simulink library "NCS_Library"  (R2019a)
settings: Solver=VariableStepAuto  StartTime=0.0  StopTime=10.0  RelTol=1e-3
values from neighbouring files (symbols this model uses):
  A = 10    [Parameter.m]
  band = 100000000    [Parameter.m]
  BER = 0    [Parameter.m]
  c = 5000000    [Parameter.m]
  c1 = 4.33    [Parameter.m]
  c2 = 3.16    [Parameter.m]
  CAN2EthernetDelay = 0.000    (= 0)    [Parameter.m]
  cR = 1.5*10^-3    (= 0.0015)    [Parameter.m]
  cw = (cwE * 2 + cwM * (nW_ges-2))/nW_ges    (= 0.1475)    [Parameter.m]
  cwE = 0.35    [Parameter.m]
  cwM = 0.08    [Parameter.m]
  Cycle_Controller = 0    [Parameter.m]
  CyclePLC = 24/1000    (= 0.024)    [Parameter.m]
  d = 800000    [Parameter.m]
  Dr = 0.92    [Parameter.m]
  Ethernet2CANDelay = 0.005    [Parameter.m]
  F_konst = 70892    [Parameter.m]
  FA = 100000    [Parameter.m]
  FB_WB_max = 10000    [Parameter.m]
  FBel_an = iG*nG*F_KZmax*nBan*R_mR/(Dr/2)    (= 28197.4297239)    [Parameter.m]
  FBel_frei = iG*nG*F_KZmax*nBfrei*R_mW/(Dr/2)    (= 29270.6882948)    [Parameter.m]
  Fmaxdyn = 300000    [Parameter.m]
  g = 9.81    [Parameter.m]
  i = 0    [Parameter.m]
  J = 1/2*mA*(Dr/2)^2    (= 158.7)    [Parameter.m]
  k1 = 0.095    [Parameter.m]
  k2 = 9.26/3.6    (= 2.57222222222)    [Parameter.m]
  k3 = 4.63/3.6    (= 1.28611111111)    [Parameter.m]
  mges = 58000    [Parameter.m]
  mu = [mu1 mu2]    [Parameter.m]
  muBel1 = 0.42    [Parameter.m]
  muBel2 = 0.36    [Parameter.m]
  n = 0.001    [Parameter.m]
  n_Mg = 4    [Parameter.m]
  n_WB = 4    [Parameter.m]
  nA = 4    [Parameter.m]
  nBan = 2    [Parameter.m]
  nBfrei = 3    [Parameter.m]
  nM = 4    [Parameter.m]
  nW_an = 4    [Parameter.m]
  P_max = 8200000    [Parameter.m]
  Q = 10    [Parameter.m]
  r_reib = 600    [Parameter.m]
  rho = 1.08    [Parameter.m]
  rhoL = 1.225    [Parameter.m]
  Size = 8    [Parameter.m]
  slip = [s1 s2]    [Parameter.m]
  tol = 0.05    [Parameter.m]
  v00 = 100/3.6    (= 27.7777777778)    [Parameter.m]
  v_grenz = 60/3.6    (= 16.6666666667)    [Parameter.m]
  v_opt = 75/3.6    (= 20.8333333333)    [Parameter.m]
  W_opt = 0.5    [Parameter.m]
  WB = 1    [Parameter.m]
  y_opt = sqrt(W_opt)/((1+sqrt(W_opt))^2+W_opt)    [Parameter.m]
undefined symbols (not defined in the file or in its folder): BUSCapacity, CableLength, controlGate, D_dyn, D_mg, EnableBurst, EnableToF, entity, Entity_out, Gate, Gate_4, Gate_5, Gate_ACK, Gate_copy, Gate_RX, getData, gettime, I_dyn, I_mg, m, magnitude, P_dyn, P_mg, ReadAttributes, readdata, ReadData, ReadSize, sigbuilder_block, Timeout, ToB, ToF, v0, v_d, v_soll
libraries: simulink x176, $bdroot x102
(part 11 of 12)

== matlab function NCS_Library/Network/ETB/OSI Layers/IP/Simulink Function/MATLAB Function ==
  data: Source input; Destination input; MACSource output; MACDestination output
function [ MACSource, MACDestination ] = GetMAC( Source, Destination)
% This function determnines if the the destination of the entity is of
% the same consist or of a remote consist.
% If it is in a remote consist, the entity is sent to the TBN/router.
if Source(1) == Destination(1)
    MACDestination = uint16(Destination(2));
elseif Destination(1) == 100
    % Multicast
    MACDestination = uint16(200);
else
    MACDestination = uint16(99);
    % to router
end
MACSource = Source(2);
end % end function

== stateflow chart NCS_Library/Network/Gateway/Gateway1/CAN Interface/CAN Interface/Reception Control ==
  settings: enableNonTerminalStates=1
  state Process
    en:
    Port.data=S;
    send(Port);
  state [Status,Ack] = Compute(rx_id,loss,rx_rtr,rx_data,tx_id,tx_rtr,tx_data) [function]
  (default) -> Process : {S=1; Ack=0; TX_ID=-1; TX_RTR=0; TX_Data=0;}
  Process -> Process [order 1] : TX{TX_ID=TX.data.ID; TX_RTR=TX.data.RTR; TX_Data=TX.data.Data;}
  (junction 12) -> Process [order 1] : [Ack==1]{Success.data=1; send(Success);}
  (junction 12) -> Process [order 2] : [Ack==0]{ReTX.data=1; send(ReTX);}
  Process -> (junction 12) [order 2] : RX{[S,Ack]=Compute(RX.data.ID,...
      |                         RX.data.RndLoss, ...
      |                         RX.data.RTR, ...
      |                         RX.data.Data, ...
      |                         TX_ID, ...
      |                         TX_RTR, ...
      |                         TX_Data);}
  data: Status function_output; Ack function_output; rx_id function_input double size=1; loss function_input double size=1; rx_rtr function_input double size=1; rx_data function_input double size=1; tx_id function_input double size=1; tx_rtr function_input double size=1; tx_data function_input double size=1; TX input Bus: CAN_Message; RX input Bus: CAN_Message; S local; Ack local; TX_ID local; TX_RTR local; TX_Data local; Port output; Success output; ReTX output

== matlab function NCS_Library/Network/Gateway/Gateway1/CAN Interface/CAN Interface/Reception Control/Compute/MATLAB Function ==
  data: ID0 input; ACK output; RTR0 input; Data0 input; ID1 input; RTR1 input; Data1 input; Loss input
function ACK = fcn(ID0,RTR0,Data0,ID1,RTR1,Data1,Loss)
% Compare the message ID, RTR, Data fields to acknowledge a successful send

if (ID0 == ID1 && RTR0 == RTR1 && Data0 == Data1 && Loss < 1)
    ACK = 1;
else
    ACK = 0;
end

== stateflow chart NCS_Library/Network/Gateway/Gateway1/CAN Interface/Save Data/Hold Data ==
  state Init
    en: SavedData=InData;
  state Save_Data
    du: OutData=SavedData;
  state Push_Data
    en: OutData=SavedData;
  (default) -> Init
  Init -> Save_Data
  Push_Data -> Save_Data
  Save_Data -> Push_Data : [Flush==1]{SavedData=InData;}
  data: Flush input; InData input; SavedData local; OutData output

== matlab function NCS_Library/Network/Gateway/Gateway1/CAN Interface/Save Data/MATLAB Function ==
  data: refresh input; write input; Type input; Data input; M_Data output; M_Data_old input
function M_Data = SaveData (refresh, write, Type, Data, M_Data_old)
%% Init
M_Data = zeros(3,20);
M_Data(1,1) = 1;

if refresh
    % refresh matrix
else
    % save data in matrix
    M_Data = M_Data_old;
    if write && Type > 0 && Type < 3
        if M_Data(1,1) == 1
            % no data saved yet
            M_Data(Type,2) = Data;          % save data
            M_Data(1,1) = M_Data(1,1)+1;    % update length
        else
            % compare the data to write with the data already saved in the matrix
            for i=2:M_Data(1,1)+1
                if M_Data(1,i) ~= 0 || M_Data(2,i) ~= 0 || M_Data(3,i) ~= 0
                    % there is data at current position
                    if M_Data(Type,i) == Data
                        % data on current position is data to write
                        break;  % data already saved in Ethernet entity
                    end
                else
                    M_Data(Type,i) = Data;          % save data
                    M_Data(1,1) = M_Data(1,1)+1;    % update length
                    break;  % finished
                end
            end % endfor
        end
    end %endif write
end % endif refresh
end % function

== matlab function NCS_Library/Network/ETB/OSI Layers/IP/Simulink Function1/MATLAB Function ==
  data: Address input; Route output; Source input; Destination input; SN input
function Route = Addressing(Address, Source, Destination, SN)
%% This function determines if the incoming entity is a mulitcast of a subscribed node
% It checks if there is a multicast and if the source is a subscribed node.
% Depending on that, the route is chosen.
%% Init
Route = uint8(2);
s = size(SN);
%% get route
if Destination(1) < 100
    % invalid address
    Route = uint8(2);   % discard
elseif Destination(1) == Address(1)
    if Destination(2) == 200
        % Broadcast to Consist
        Route = uint8(2);
        for i=1:s(2)
            if Source(1) == SN(i,1) && Source(2) == SN(i,2) && Source(3) == SN(i,3) && Source(4) == SN(i,4)
                % subscribed to node
                Route = uint8(1);  
                break;
            end
        end
    elseif Destination(4) == Address(4)
            Route = uint8(1);  % set route
    else
        Route = uint8(2);   % discard
    end
elseif Destination(1) == 100
    % Multicast
    Route = uint8(2);
    for i=1:s(2)
        if Source(1) == SN(i,1) && Source(2) == SN(i,2) && Source(3) == SN(i,3) && Source(4) == SN(i,4)
            % subscribed to node
            Route = uint8(1);  
            break;
        end
    end
else
    Route = uint8(2);   % discard
end % endif
end % end function

== matlab function NCS_Library/Network/ETB/OSI Layers/TRDP PD/Simulink Function1/MATLAB Function2 ==
  data: msgType input; ReplyAddress input; DestinationPull output
function DestinationPull = Receive(msgType, ReplyAddress)

DestinationPull = uint16( [0 0 0 0] );

if msgType == 11
    % Request
    DestinationPull = ReplyAddress;
end
        
end % end function

== matlab function NCS_Library/Network/ETB/OSI Layers/TRDP PD/Simulink Function/MATLAB Function ==
  data: Data input; Data_edited output; msgType input
function Data_edited = EditData(Data, msgType)
%% Edit Data
% Replace data with zero in the case of a request or an error.

if msgType == 11 || msgType == 14
    Data_edited = zeros(3, 20);
else
    Data_edited = Data;
end

end % end of function

== matlab function NCS_Library/Network/ETB/OSI Layers/SDTv2/MATLAB Function ==
  data: T_signal input; msgType input; y output; T_tx input
function y = fcn(T_signal, msgType, T_tx)

if msgType == 11
    y = T_signal;
else
    y = T_tx;
end
end

== matlab function NCS_Library/Network/ETB/OSI Layers/SDTv2/Simulink Function1/MATLAB Function ==
  data: SSC_received output; SSC_last input; SSC input; Route output
function [ SSC_received , Route]= Check( SSC_last, SSC)
%% Check the SSC of the VDP
% This functions checks the SSC of an arriving VDP. If the SSC is greater
% or equal to SSC of the last fresh VDP received the VDP is valid. If it is
% greater than the last, the VDP is fresh and its SSC is saved.

Route = uint8(2); % discard for default
SSC_received = SSC_last;

if SSC > SSC_last
    Route = uint8(1);
    SSC_received = SSC;
elseif SSC == 0
    % Init
    Route = uint8(1);
end

== matlab function NCS_Library/Network/ETB/Controller Interface/Parameter/MATLAB Function ==
  data: In1 input; In2 input; msgType output; In3 input; In4 input
function msgType = GetmsgType(In1, In2, In3, In4)

In = [In1 In2 In3 In4];

n = length(In);
msgType = uint8(zeros(n,1));   % Init

for i=1:n
    if In(i) == 1
        % Push Data
        Type = 13;
    else
        Type = 0;
    end
    msgType(i) = uint8(Type);
end
end % end function

== matlab function NCS_Library/Network/ETB/OSI Layers/SDTv2/Get Phase/MATLAB Function ==
  data: Phase_previous input; LSC input; Phase output; Contraction input; Init input
function Phase = Get_SDTv2_Phase(Phase_previous, LSC, Contraction, Init)
%% This function determines the phase of the SDTv2
% Phase 0: no inital VDP sampled
% Phase 1: Safe
% Phase 2: Sink-Time error
% Phase 3: Contraction
%% Set Phase
Phase = Phase_previous;

switch Phase
    case 0
        % No received inital VDP
        if Init
            Phase = 1;
        else
            Phase = 0;
        end
    case 1
        % Safe communication
        if LSC
            Phase = 2;
        elseif Contraction
            Phase = 3;
        else
            Phase = 1;
        end
    case 2
        % Lost of safe communication
        if ~LSC
            Phase = 1;
        end
    case 3
        if ~Contraction
            Phase = 1;
        end
    otherwise
        Phase = 10;
end
end % end function

== matlab function NCS_Library/Network/ETB/Controller Interface/Parameter/MATLAB Function1 ==
  data: Destination output; Actuators input; Sensors input; Subscribe output
function [ Destination, Subscribe]= AddMatrices(Actuators, Sensors)

Destination = [ Actuators zeros(length(Actuators),2)];
Sensors = [ Sensors zeros(length(Sensors),2)];
Subscribe = [Sensors; Destination];
end % end function

== matlab function NCS_Library/Network/ETB/OSI Layers/Application/Edit Paramter/MATLAB Function ==
  data: UDP input; U input; y output
function y = fcn(UDP, U)
% Select corresponding line of the matrix U containing the addresses of the
% actuators. The used address is in the line equals to the UDP-Port.
y = U(UDP,:);

end % end function

== matlab function NCS_Library/Network/ETB/Subsystem2/Routing Layer/Logic 3/Simulink Function1/MATLAB Function ==
  data: MACDestination output; S1 input; Route output; S2 input; S3 input; Destination input; RT input
function [MACDestination, Route] = Routing( S1, S2, S3, Destination, RT)
%%
%
%% Init
Route = 1;
if Destination(1) == 100
    % Multicast
    Route = 4;
    MACDestination = uint16(200);
else
    for i=1:length(RT)
        if Destination(1) == RT(i,1)
            % found entry in routing table
            break;
        end
    end % end for

    if RT(i,1) == S1 || ( RT(i,1) == S1 && S1 > 0)
        Route = 1;
    elseif RT(i,1) == S2 || (RT(i,1) == S2 && S2 > 0)
        Route = 2;
    elseif RT(i,1) == S3 || (RT(i,1) == S3 && S3 > 0)
        Route = 3; 
    end

    if Destination(1) == S1 || Destination(1) == S2 || Destination(1) == S3
        % To local node
        MACDestination = Destination(2);
    else
        % To next Router
        MACDestination = uint16(RT(i,2));
    end % endif
end

end % end function

== matlab function NCS_Library/Network/ETB/OSI Layers/Application/Edit Paramter/MATLAB Function1 ==
  data: Port input; Value output; In input
function Value = Select(Port, In)
%% Select Value depending on UDP port

s = size(In);
if s(1) >= Port
    Value = In(Port,:);
else
    Value = In(1,:);
end
end % end function

== matlab function NCS_Library/Network/ETB/OSI Layers/Application/Edit Paramter/MATLAB Function2 ==
  data: Port input; Value output; In input
function Value = Select(Port, In)
%% Select Value depending on UDP port

s = size(In);
if s(1) >= Port
    Value = In(Port,:);
else
    Value = In(1,:);
end
end % end function

== matlab function NCS_Library/Network/ETB/OSI Layers/Application/Edit Paramter/MATLAB Function3 ==
  data: Port input; Value output; In input
function Value = Select(Port, In)
%% Select Value depending on UDP port

s = size(In);
if s(1) >= Port
    Value = In(Port,:);
else
    Value = In(1,:);
end
end % end function

== matlab function NCS_Library/Network/ETB/OSI Layers/MAC Controller/CSMA//CD Entry/MATLAB Function ==
  data: n input; collision output; collision input
function collision = DetectCollisionEntry(n, collision)

if collision
    % packet already collided
    % hence nothing left to do
else
    if n > 1
        % more than one packet in bus
        collision = uint8(2);
    else
        collision = uint8(0);
    end
end
end % end function

== matlab function NCS_Library/Network/ETB/Subsystem2/Routing Layer/Logic 2/Simulink Function1/MATLAB Function ==
  data: MACDestination output; S1 input; Route output; S2 input; S3 input; Destination input; RT input
function [MACDestination, Route] = Routing( S1, S2, S3, Destination, RT)
%%
%
%% Init
Route = 1;
if Destination(1) == 100
    % Multicast
    Route = 4;
    MACDestination = uint16(200);
else
    for i=1:length(RT)
        if Destination(1) == RT(i,1)
            % found entry in routing table
            break;
        end
    end % end for

    if RT(i,1) == S1 || ( RT(i,1) == S1 && S1 > 0)
        Route = 1;
    elseif RT(i,1) == S2 || (RT(i,1) == S2 && S2 > 0)
        Route = 2;
    elseif RT(i,1) == S3 || (RT(i,1) == S3 && S3 > 0)
        Route = 3; 
    end

    if Destination(1) == S1 || Destination(1) == S2 || Destination(1) == S3
        % To local node
        MACDestination = Destination(2);
    else
        % To next Router
        MACDestination = uint16(RT(i,2));
    end % endif
end

end % end function

== matlab function NCS_Library/Network/ETB/Subsystem2/Routing Layer/Logic 1/Simulink Function1/MATLAB Function ==
  data: MACDestination output; S1 input; Route output; S2 input; S3 input; Destination input; RT input
function [MACDestination, Route] = Routing( S1, S2, S3, Destination, RT)
%%
%
%% Init
Route = 1;
if Destination(1) == 100
    % Multicast
    Route = 4;
    MACDestination = uint16(200);
else
    for i=1:length(RT)
        if Destination(1) == RT(i,1)
            % found entry in routing table
            break;
        end
    end % end for

    if RT(i,1) == S1 || ( RT(i,1) == S1 && S1 > 0)
        Route = 1;
    elseif RT(i,1) == S2 || (RT(i,1) == S2 && S2 > 0)
        Route = 2;
    elseif RT(i,1) == S3 || (RT(i,1) == S3 && S3 > 0)
        Route = 3; 
    end

    if Destination(1) == S1 || Destination(1) == S2 || Destination(1) == S3
        % To local node
        MACDestination = Destination(2);
    else
        % To next Router
        MACDestination = uint16(RT(i,2));
    end % endif
end

end % end function

== stateflow chart NCS_Library/Network/Gateway/Gateway2/Ethernet Interface/Subsystem4/Chart ==
  state Buffer_empty
    en: n=0;
    en: Push = 0;
  state Buffer_full
    du: Push=0;
  (default) -> Buffer_empty
  Buffer_full -> Buffer_empty [order 4] : [n==0]
  Buffer_empty -> Buffer_full [order 1] : [NEW>0]{n=n+NEW;}
  Buffer_empty -> Buffer_full [order 2] : [n>0]
  Buffer_full -> Buffer_full [order 1] : [NEW>0&&TIME==1]{n=n+NEW-1;}
  Buffer_full -> Buffer_full [order 3] : [TIME==1]{n=n-1;Push=1;}
  Buffer_full -> Buffer_full [order 2] : [NEW>0]{n=n+NEW}
  data: TIME input; n local; NEW input; Push output

== matlab function NCS_Library/Network/ETB/Cable/MATLAB Function ==
  data: Cable input; NVP output
function NVP = GetNVP(Cable)

switch Cable
    case 1
        NVP = 0.7;
    otherwise
        NVP = 1;
end
end % end of function

== matlab function NCS_Library/Network/ETB/OSI Layers/TRDP PD/Transmit ==
  data: Buffer_old input; Buffer output; lst input; Pull input; msgTypeReply input; DestinationReply input; Cycle input; Push input; SDTv2 input; msgTypePush input; DestinationPush input; lst_old output; msgType output; Destination output
function [ Buffer, lst_old, msgType, Destination ]  = Buffer( Buffer_old, lst, Pull, msgTypeReply, DestinationReply, Cycle, Push, SDTv2, msgTypePush, DestinationPush)
%% Init
msgType = uint8(0);
Destination = uint16( [0 0 0 0] );
Buffer = zeros(100,5);
lst_old = 0;
s = [0 0];

if SDTv2 == 1
    n_msg = 3;
else
    n_msg = 1;
end

%% Handle Input
Buffer = Buffer_old;
if Push == 1
    lst = lst+1;
    Buffer(lst,1) = double(msgTypePush);
    Buffer(lst,2:5) = double(DestinationPush); 
end % end if

if Push == 2
    lst = lst+1;
    Buffer(lst,1) = double(msgTypePush);
    Buffer(lst,2:5) = double(DestinationPush); 
end % end if

%--------------------------
% Pull
%--------------------------
if Pull
    lst = lst+1;
    Buffer(lst,1) = double(msgTypeReply);
    Buffer(lst,2:5) = double(DestinationReply);    
end

%% Generate Message
if Cycle
    % Transmit
    msgType = uint8(Buffer(1,1));
    Destination = uint16(Buffer(1,2:5));

    % Update Buffer
    if lst == 0
        lst_old = 0;
    elseif lst == 1
        lst_old = 0;
        Buffer = zeros(100,5);
    else
        lst_old = lst-1;
        Buffer(1:lst-1,:) = Buffer(2:lst,:);   
    end
end

end % end function

== matlab function NCS_Library/Network/ETB/ED/User Interface/MATLAB Function ==
  data: u input; msgType output
function msgType = GetmsgType(u)

switch u
    case 1
        msgType = 11;
    case 2
        msgType = 13;
    case 3
        msgType = 13;
    otherwise
        msgType = 0;
end
end % end function

== matlab function NCS_Library/Network/ETB/OSI Layers/TRDP PD/MATLAB Function1 ==
  data: Event input; Time input; T_tx input; Push output; msgType input
function Push = Push(Event, Time, T_tx, msgType)
Push = 0;

if T_tx == 0
    % discrete
    if msgType && Event
        Push = 2;
    end
else
    % continuous
    if msgType && Time
        Push = 1;
    end
end
end % end function

== matlab function NCS_Library/Network/ETB/OSI Layers/TRDP PD/Simulink Function1/MATLAB Function ==
  data: Reply input; Address output; Source input
function Address = GetAddress(Reply, Source)
Address = Reply;
if Reply(1) == 0
    Address = Source;
end

== stateflow chart NCS_Library/Network/CAN/CAN Node 1/Reception Control ==
  settings: enableNonTerminalStates=1
  state Process
    en:
    Port.data=S;
    send(Port);
  state [Status,Ack] = Compute(rx_id,loss,rx_rtr,rx_data,tx_id,tx_rtr,tx_data) [function]
  (default) -> Process : {S=1; Ack=0; TX_ID=-1; TX_RTR=0; TX_Data=0;}
  Process -> Process [order 1] : TX{TX_ID=TX.data.ID; TX_RTR=TX.data.RTR; TX_Data=TX.data.Data;}
  (junction 12) -> Process [order 1] : [Ack==1]{Success.data=1; send(Success);}
  (junction 12) -> Process [order 2] : [Ack==0]{ReTX.data=1; send(ReTX);}
  Process -> (junction 12) [order 2] : RX{[S,Ack]=Compute(RX.data.ID,...
      |                         RX.data.RndLoss, ...
      |                         RX.data.RTR, ...
      |                         RX.data.Data, ...
      |                         TX_ID, ...
      |                         TX_RTR, ...
      |                         TX_Data);}
  data: Status function_output; Ack function_output; rx_id function_input double size=1; loss function_input double size=1; rx_rtr function_input double size=1; rx_data function_input double size=1; tx_id function_input double size=1; tx_rtr function_input double size=1; tx_data function_input double size=1; TX input Bus: CAN_Message; RX input Bus: CAN_Message; S local; Ack local; TX_ID local; TX_RTR local; TX_Data local; Port output; Success output; ReTX output

== matlab function NCS_Library/Network/CAN/CAN Node 1/Reception Control/Compute/MATLAB Function ==
  data: ID0 input; ACK output; RTR0 input; Data0 input; ID1 input; RTR1 input; Data1 input; Loss input
function ACK = fcn(ID0,RTR0,Data0,ID1,RTR1,Data1,Loss)
% Compare the message ID, RTR, Data fields to acknowledge a successful send

if (ID0 == ID1 && RTR0 == RTR1 && Data0 == Data1 && Loss < 1)
    ACK = 1;
else
    ACK = 0;
end

== matlab function NCS_Library/Network/Gateway/Gateway1/Ethernet Interface/Buffer ==
  data: updatedBuffer input; Push input; Buffer output; Data input; data output
function [Buffer, data] = GatewayBuffer(updatedBuffer, Push, Data)

%% Init
Buffer = zeros(3,100);
FIN = 0;

Buffer = updatedBuffer;
%% Write to buffer
for i=2:Data(1,1)
    for j=1:length(Buffer)
        if Buffer(1,j) == 0 && Buffer(2,j) == 0 && Buffer(3,j) == 0
            % free position
            % save data
            Buffer(:,j) = Data(:,i);
            break;

        elseif Data(1,i) == Buffer(1,j) && Data(2,i) == Buffer(2,j) && Data(3,i) == Buffer(3,j)
            % data already in buffer
            FIN = 1;
            break;
        end
    end % end for
    
    if FIN
        % data already in buffer
        break;
    end
end % end for

%% Push
if Push
    % Read from buffer
    data = Buffer(:,1);

    % Udpdate buffer
    Buffer(:,1:length(Buffer)-1) = Buffer(:,2:length(Buffer));
else
    data = [0;0;0];
end

end % end function

== matlab function NCS_Library/Network/Gateway/Gateway1/Ethernet Interface/User Interface/MATLAB Function ==
  data: u input; msgType output
function msgType = GetmsgType(u)

switch u
    case 1
        msgType = 11;
    case 2
        msgType = 13;
    case 3
        msgType = 13;
    otherwise
        msgType = 0;
end
end % end function

== matlab function NCS_Library/Network/Gateway/Gateway1/Ethernet Interface/User Interface/MATLAB Function1 ==
  data: u input; y output
function y = fcn(u)

m = length(u);
ADD = zeros(m,2);
y = [u ADD];

== stateflow chart NCS_Library/Network/ETB/Subsystem2/Routing Table/Get Routing Table/Router Control ==
  state Start
    en: Tx=1; Init =1;
  state Init
    en: Tx=0;
  state Failure
    Tx=0;
  state SendFailure
    Tx=1;
  state Idle
    en: Tx=0; Init=0;
  state Refresh
    en: Tx=1; Init=1;
  (default) -> Start
  Start -> Init
  Init -> Idle : [FIN==1]
  Idle -> Refresh [order 1] : [Refresh==1]
  SendFailure -> Failure
  Idle -> SendFailure [order 2] : [Failed==1]
  Refresh -> Idle : [FIN==1]
  data: Refresh input; Failed input; FIN input; Tx output; Init output

== matlab function NCS_Library/Network/ETB/Cable/Simulink Function/MATLAB Function ==
  data: Time input; Source input; SEQ input; BER input; CheckBit output
function CheckBit = BitError(Time, Source, SEQ, BER)
%% calculate checksum
% This function computes a random number using the current simulation time, 
% NodeID and the SEQ of the current entity. If this random number is 
% smaller than the bit-error-rate (BER), than a bit-error occurs, thus the 
% checksum is set to zero. Otherwise the checksum remains one.
%%
% define settings for random number generator
rng(10000*Time+double(Source(1))+double(Source(2))+double(Source(3))+double(Source(4))+SEQ);
random = rand(1);               % generate random number
if random <= BER
    % bit-error
    CheckBit = uint8(0);
else
    % ok
    CheckBit = uint8(1);
end
end % function

== matlab function NCS_Library/Network/ETB/OSI Layers/TRDP PD/Enabled Subsystem1/MATLAB Function ==
  data: msgType input; msgTypeReply output
function msgTypeReply = SetMessageTypeReply(msgType)
%% 
% Sets the message type to 12 (Reply), if arequest was sampled. Else the
% msgType is set to 0, so no entity is created.

if msgType == 11
    msgTypeReply = uint8(12);
else
    msgTypeReply = uint8(0);
end

== stateflow chart NCS_Library/Controller/Logic/Braking Controller/Steuerung ==
  state konstante_Fahrt
    en: status = 1;
  state Leerlauf
    en: status = 0;
  state Betriebsbremsung
    en: status = 2;
  state Schnellbremsung
    en: status = 3;
  konstante_Fahrt -> Leerlauf [order 3] : [fahrst == 0]
  Leerlauf -> konstante_Fahrt [order 1] : [fahrst == 1]
  Betriebsbremsung -> konstante_Fahrt [order 3] : [fahrst == 1 || v <= v_soll]
  konstante_Fahrt -> Schnellbremsung [order 1] : [fahrst == 3]
  konstante_Fahrt -> Betriebsbremsung [order 2] : [fahrst == 2 && v > v_soll]
  (default) -> Leerlauf
  Betriebsbremsung -> Leerlauf [order 1] : [fahrst == 0]
  Leerlauf -> Betriebsbremsung [order 2] : [fahrst == 2 &&  v > v_soll]
  Schnellbremsung -> Leerlauf : [fahrst == 0]
  Leerlauf -> Schnellbremsung [order 3] : [fahrst == 3]
  Betriebsbremsung -> Schnellbremsung [order 2] : [fahrst == 3]
  data: fahrst input; emerg input; status output; v_soll input; v input

== stateflow chart NCS_Library/Network/Applications/Subsystem/Burst Control ==
  state Idle
    en: Burst=0;
  state Burst
    en: Burst=1;
  state Idle2
    en: Burst=0
  (default) -> Idle
  Idle -> Burst : [Enable==1 && ToF==1]
  Burst -> Idle2
  data: Burst output; ToF input; Enable input

== matlab function NCS_Library/Network/ETB/Ethernet_2-port_Switch/Determine Port_N/MATLAB Function ==
  data: Anew output; Destination input; y output; Source input; A input; B input; maxn input
function [Anew,y] = findport(Destination,Source,A,B,maxn)

for n=1:1:maxn
    if A(n)==Source
        break
    end
end
saven = n - 1
for n=1:1:saven
    A(n+1)=A(n);
end
A(1) = Source;

n = 1;
while n <= maxn
    if A(n) == Destination
        break
    end
    n = n + 1;
end
if n > maxn
    n = 1;
    while n <= maxn
        if B(n)==Destination
            break
        end
        n = n + 1;
    end
    if n > maxn
            y = 2;
    else
            y = 1;
    end
else
    y = 0;
end
Anew = A;
end

== stateflow chart NCS_Library/Network/ETB/OSI Layers/TRDP Timeout/TRDP Timeout ==
  state Idle
  state ReStart_Timer
    en: Timeout=0; Time=Clock;
  state Timeout
    en: Timeout=1;
  (default) -> Idle
  Idle -> ReStart_Timer : [Reception]
  ReStart_Timer -> ReStart_Timer [order 2] : [Reception]
  Timeout -> ReStart_Timer : [Reception]
  ReStart_Timer -> Timeout [order 1] : [Clock-Time>Timeout_Value]
  data: Reception input; Clock input; Timeout_Value input; Time local; Timeout output

== matlab function NCS_Library/Network/ETB/ED/User Interface/MATLAB Function1 ==
  data: u input; y output
function y = fcn(u)

m = length(u);
ADD = zeros(m,2);
y = [u ADD];

== matlab function NCS_Library/Network/ETB/OSI Layers/TRDP PD/Detect Event/DetectEvent ==
  data: U input; Change output; Memory input; M output
function [Change, M] = DetectChange(U, Memory)

Change = 0;
M = U;
size_U = size(U);

for i=1:size_U(1)
    for j=1:size_U(2)
        if U(i,j) ~= Memory(i,j)
            Change = 1;
            break;
        end
    end
end

end % end function

== matlab function NCS_Library/Network/ETB/Subsystem2/Routing Table/Get Routing Table/Compute Routing Table/MATLAB Function ==
  data: ID input; RM input; RT output
function RT = getRT(ID, RM)
%% Init
ERROR = [0 0];
RT = zeros(1000,4);
r = 1;              % row index of RT
subnets = zeros(5,1);

%% get routing table
for i=2:RM(1,1) 
        FIN = 0;                            % reset FIN
        path = zeros(100,3);        % inititlize path
        path(1,1) = 1;                      % initilize search-path index
        % path(:,2) = zeros(length(path),1); % resets counter
        
        if RM(i,2) > 100                    % check if in the second column is a subnet
            
            % find subnets to router
            t = 0; % Init
            for s=2:RM(1,1)
                if RM(s,1) == ID && RM(s,2) > 100
                    % line contains subnet connected to own router
                    t = t+1;                % update t
                    subnets(t) = RM(s,2);   % save subnet                
                end
            end
            
            while FIN == 0
                % Init
                subnet = 0;             % reset subnet
                FIN = 1;
                hops = 1;                       % set hops
                p = path(1,1);                  % save start of new path
                current = RM(i,1);              % set starting position
                next = current;
                while next ~= ID                % as long as we didn't reach our router -> DO
                    %% updates for new hop
                    current = next;           
                    % Init
                    k_last = length(path);      % set k_last                   
                    %%  find next hop
                    for j=2:RM(1,1)
                        if RM(j,2) == current                           
                            for k=path(1):-1:1
                                if RM(j,3) == path(k,1)
                                    % found hop
                                    break;
                                end
                            end
                            % check if hop ends at own router
                            OWN = 0;
                            for u=1:t
                                if subnets(u) == RM(j,3)
                                    % next hop is to own router
                                    OWN = 1;
                                    break;
                                end
                            end
                            % check case
                            if k == 1
                                % hop was never done before
                                FIN = 0;
                                next = RM(j,1);         % save next router
                                subnet = RM(j,3);       % save next hop
                                break;                  % found next hop
                            else
                                if OWN
                                    % next hop is to own router
                                    next = RM(j,1);         % save next router
                                    subnet = RM(j,3);       % save next hop
                                    break;                  % found next hop
                                else
                                    if k < k_last
                                        % hop is the oldest hop
                                        next = RM(j,1);         % save next router
                                        subnet = RM(j,3);       % save next hop
                                        k_last = k;             % update k_last
                                    end
                                end                                
                            end                                       
                        end
                    end % end for
                    
                    %% evaluate next hop
                    % Init
                    RST = 0;
                    STR = 0;
                    q = 1;
                    % check if starting router is reached
                    if next == RM(i,1)
                        STR = 1;
                    else
                        % check if router was used before in current path
                        for q=p:path(1,1)
                            if path(q,2) == next
                                RST = 1;
                                break;
                            end
                        end
                    end
                    
                    % update hops
                    if ~RST && ~STR
                        % new router
                        hops = hops+1;      % new hop                        
                    end
                    if RST
                        % router already used
                        hops = path(q,3);   % reset hops
                    end
                    if STR
                        % next hop reaches start router
                        hops = 1;           % reset hops
                    end
                                        
                    % save hop in path
                    path(1,1) = path(1,1)+1;    % update number of rows
                    path(path(1),1) = subnet;   % save hop in path
                    path(path(1),2) = next;     % save next router
                    path(path(1),3) = hops;     % save the number of hops

                    if current == next      % no connected router
                       ERROR = [ 1, ID ];   % throw error
                       break;           
                    end           
                end % end of search for one path
                
                % save path in path
                path(1) = path(1)+1;    % update number of rows
                path(path(1))= 0;       % fill in zero 

                % save entry in routing table
                RT(r,1) = RM(i,2);              % save subnet ID
                RT(r,2) = current;              % save next router
                RT(r,3) = subnet;               % save next subnet    
                RT(r,4) = hops;                 % save number of hops

                r = r+1;                        % go to next row of routing table
            end % end of search for all paths
        
        end % end if

        % catch
        if ERROR(1,1) ~= 0
            break;  % stop loop
        end
end % end of for-loop over routing matrix

%% edit routing table
for m=1:r
    for n=1:r
        if RT(m,1) == RT(n,1) && m~=n && RT(m,4) <= RT(n,4)
            % two lines have the address the same subsystem
            % and first line has less hops
            RT(n,:) = [0 0 0 0];  % replace second line with zeros            
        end
    end
end

for m=1:r
    if RT(m,1) == 0                 % check if there is a dead line
        for n=m+1:r
            if RT(n,1) ~= 0
                RT(m,:) = RT(n,:);  % save line instead of dead line
                RT(n,:) = [0 0 0 0];  % delete line
                break;
            end
        end
    end
end

end % end of function

== matlab function NCS_Library/Network/ETB/Ethernet_3-port_switch/Determine Port_R/MATLAB Function ==
  data: Anew output; Destination input; y output; Source input; A input; B input; C input; maxn input
function [Anew, y] = findport(Destination,Source,A,B,C,maxn)

for n=1:1:maxn
    if A(n)==Source
        break
    end
end
saven = n - 1
for n=1:1:saven
    A(n+1)=A(n);
end
A(1) = Source;

n = 1;
while n <= maxn
    if A(n) == Destination
        break
    end
    n = n+1;
end
if n > maxn
    n = 1; 
    while n <= maxn
        if B(n)==Destination
            break
        end
        n = n + 1;
    end
    if n > maxn
        n = 1;
        while n <= maxn
            if C(n) == Destination
                break
            end
            n = n + 1;
        end
        if n > maxn
            y = 3;
        else
            y = 2;
        end
    else
        y = 1;
    end
else
    y = 0;
end
Anew = A;
end

== matlab function NCS_Library/Network/ETB/Subsystem2/Routing Table/Get Routing Table/Simulink Function1/Compute local routing matrix ==
  data: ID input; R_local output; s input
function R_local = InitR(ID, s)
%% Init R
R_local = zeros(10,2);
R_local(1,1) = 1;

%% Set connected subsystems
% get number of values
for i=1:length(s)
    if s(i) ~= 0
        R_local(1,1) = R_local(1,1)+1;          % update lst
        R_local(R_local(1,1),:) = [ double(ID) s(i) ];  % write data in lst
        
    end
end   

end % end of function

== stateflow chart NCS_Library/Network/Applications/TRDP Timeout/Chart ==
  state Init
    en: Valid=1;
  state Start_Timer
    en: Time = currentTime;
    en: Valid = 1;
  state Timeout
    en: Valid = 0;
  (default) -> Init
  Init -> Start_Timer : [Restart_Timer]
  Start_Timer -> Start_Timer [order 1] : [Restart_Timer]
  Start_Timer -> Timeout [order 2] : [currentTime-Time>=Timeout]
  Timeout -> Start_Timer : [Restart_Timer]
  data: Timeout input; Valid output; Restart_Timer input; currentTime input; Time local

== matlab function NCS_Library/Network/ETB/Subsystem2/Routing Table/Get Routing Table/Compute routing matrix RM/MATLAB Function ==
  data: state_out output; FIN output; RM_global output; state input; RM_in input; RM_old input
function [state_out, FIN, RM_global] = getRM(state, RM_in, RM_old)
%% Init
FIN = 0;
state_out=1;
RM_global = zeros(1000,3);
%%
switch state
    case 1 % Idle
        if RM_in(1,1) ~= 0
            % handling of first data
            for m=2:RM_in(1,1)
                    RM_global(RM_global(1,1)+m,1) = RM_in(m,1);
                    RM_global(RM_global(1,1)+m,2) = RM_in(m,2);
            end

            RM_global(1,1) = RM_global(1,1) + RM_in(1,1);   % update lst
            state_out = 2;                                  
        end
    case 2  % Do
        state_out = 2;  % set state for next step
        RM_global = RM_old;     % update R
        
        % handle input
         for k=2:RM_global(1,1)
            if RM_global(k,1) == RM_in(2,1)     % already got this router
                     state_out = 3;     % finished
                     break
             end
         end

         if state_out == 2    
             % new input
             for m=2:RM_in(1,1)
                RM_global(RM_global(1,1)+m-1,1) = RM_in(m,1);
                RM_global(RM_global(1,1)+m-1,2) = RM_in(m,2);
             end
            
            RM_global(1,1) = RM_global(1,1) + RM_in(1,1)-1;   % update lst
                

         end % end of handling new input
      
    case 3 % Get connections
        RM_global = RM_old;      % update RM
        lst = RM_global(1,1);   % save current lst
        
        for i=2:lst
            for j=2:lst
                if RM_global(i,2) == RM_global(j,2) && RM_global(i,1) ~= RM_global(j,1)
                    % two different routers are connected to the same subnet
                    RM_global(1,1) = RM_global(1,1)+1;                                              % update lst
                    RM_global(RM_global(1,1),:) = [ RM_global(i,1) RM_global(j,1) RM_global(i,2) ]; % write new line
                    break;                                                                          % finished
                end
            end
            
        end
        state_out = 4;
        
    case 4  % Finished
        RM_global = zeros(1000,3);  % Reset RM
        state_out = 1;  % Go back to Idle
        FIN = 1;
end

end % end function

== matlab function NCS_Library/Network/ETB/Subsystem2/Routing Table/Get Routing Table/Simulink Function2/MATLAB Function1 ==
  data: R_local input; Header output double
function Header  = ReadHeader(R_local)

Header = R_local(1,1);

end % end of function

== matlab function NCS_Library/Network/ETB/ED/User Interface/Subsystem2/MATLAB Function ==
  data: u input; y output
function y = fcn(u)

y = uint16( zeros(4,1) );
y(1) = u(1);
y(2) = u(2);

== matlab function NCS_Library/Network/ETB/Burst Device/MATLAB Function ==
  data: u input; msgType output
function msgType = GetmsgType(u)

switch u
    case 1
        msgType = 11;
    case 2
        msgType = 13;
    case 3
        msgType = 13;
    otherwise
        msgType = 0;
end
end % end function

== stateflow chart NCS_Library/Controller/Cookie/Braking Controller/Steuerung ==
  state konstante_Fahrt
    en: status = 1;
  state Leerlauf
    en: status = 0;
  state Betriebsbremsung
    en: status = 2;
  state Schnellbremsung
    en: status = 3;
  konstante_Fahrt -> Leerlauf [order 3] : [fahrst == 0]
  Leerlauf -> konstante_Fahrt [order 1] : [fahrst == 1]
  Betriebsbremsung -> konstante_Fahrt [order 3] : [fahrst == 1 || v <= v_soll]
  konstante_Fahrt -> Schnellbremsung [order 1] : [fahrst == 3]
  konstante_Fahrt -> Betriebsbremsung [order 2] : [fahrst == 2 && v > v_soll]
  (default) -> Leerlauf
  Betriebsbremsung -> Leerlauf [order 1] : [fahrst == 0]
  Leerlauf -> Betriebsbremsung [order 2] : [fahrst == 2 &&  v > v_soll]
  Schnellbremsung -> Leerlauf : [fahrst == 0]
  Leerlauf -> Schnellbremsung [order 3] : [fahrst == 3]
  Betriebsbremsung -> Schnellbremsung [order 2] : [fahrst == 3]
  data: fahrst input; emerg input; status output; v_soll input; v input

== matlab function NCS_Library/Network/ETB/Burst Device/MATLAB Function1 ==
  data: u input; y output
function y = fcn(u)

m = length(u);
ADD = zeros(m,2);
y = [u ADD];

== matlab function NCS_Library/Network/ETB/Burst Device/Protocl Stack/TRDP PD/Enabled Subsystem1/MATLAB Function ==
  data: msgType input; msgTypeReply output
function msgTypeReply = SetMessageTypeReply(msgType)
%% 
% Sets the message type to 12 (Reply), if arequest was sampled. Else the
% msgType is set to 0, so no entity is created.

if msgType == 11
    msgTypeReply = uint8(12);
else
    msgTypeReply = uint8(0);
end

== matlab function NCS_Library/Network/ETB/Burst Device/Protocl Stack/TRDP PD/Simulink Function/MATLAB Function ==
  data: Data input; Data_edited output; msgType input
function Data_edited = EditData(Data, msgType)
%% Edit Data
% Replace data with zero in the case of a request or an error.

if msgType == 11 || msgType == 14
    Data_edited = zeros(3,20);
else
    Data_edited = Data;
end

end % end of function

== stateflow chart NCS_Library/Network/CAN/CAN Node 3/Reception Control ==
  settings: enableNonTerminalStates=1
  state Process
    en: Port.data=S;
    send(Port);
  state Status = Receive(rx_id,rx_loss) [function]
  state Ack = Acknowledge(ack_id,ack_loss,ack_rtr,ack_data,tx_id,tx_rtr,tx_data) [function]
  (default) -> Process : {S=1; Ack=0; TX_ID=-1; TX_RTR=0; TX_Data=0;}
  Process -> Process [order 2] : RX{S = Receive(RX.data.ID,RX.data.RndLoss);}
  Process -> Process [order 1] : TX{TX_ID=TX.data.ID; TX_RTR=TX.data.RTR; TX_Data=TX.data.Data;}
  (junction 12) -> Process [order 1] : [Ack==1]{Success.data=1; send(Success);}
  (junction 12) -> Process [order 2] : [Ack==0]{ReTX.data=1; send(ReTX);}
  Process -> (junction 12) [order 3] : ACK{Ack=Acknowledge(ACK.data.ID,ACK.data.RndLoss,ACK.data.RTR,ACK.data.Data,TX_ID,TX_RTR,TX_Data);}
  data: Status function_output; rx_id function_input double size=1; rx_loss function_input double size=1; Ack function_output; ack_id function_input double size=1; ack_loss function_input double size=1; ack_rtr function_input double size=1; ack_data function_input double size=1; tx_id function_input double size=1; tx_rtr function_input double size=1; tx_data function_input double size=1; TX input Bus: CAN_Message; ACK input Bus: CAN_Message; RX input Bus: CAN_Message; S local; Ack local; TX_ID local; TX_RTR local; TX_Data local; Port output; Success output; ReTX output

== matlab function NCS_Library/Network/CAN/CAN Node 3/Reception Control/Acknowledge/MATLAB Function ==
  data: ID0 input; ACK output; RTR0 input; Data0 input; ID1 input; RTR1 input; Data1 input; Loss input
function ACK = fcn(ID0,RTR0,Data0,ID1,RTR1,Data1,Loss)
% Compare the message ID, RTR, Data fields to acknowledge a successful send

if (ID0 == ID1 && RTR0 == RTR1 && Data0 == Data1 && Loss < 1)
    ACK = 1;
else
    ACK = 0;
end

== stateflow chart NCS_Library/Network/CAN/CAN Node 4/Reception Control ==
  settings: enableNonTerminalStates=1
  state Process
    en: Port.data=S;
    send(Port);
  state Status = Receive(rx_id,rx_loss) [function]
  state Ack = Acknowledge(ack_id,ack_loss,ack_rtr,ack_data,tx_id,tx_rtr,tx_data) [function]
  (default) -> Process : {S=1; Ack=0; TX_ID=-1; TX_RTR=0; TX_Data=0;}
  Process -> Process [order 2] : RX{S = Receive(RX.data.ID,RX.data.RndLoss);}
  Process -> Process [order 1] : TX{TX_ID=TX.data.ID; TX_RTR=TX.data.RTR; TX_Data=TX.data.Data;}
  (junction 12) -> Process [order 1] : [Ack==1]{Success.data=1; send(Success);}
  (junction 12) -> Process [order 2] : [Ack==0]{ReTX.data=1; send(ReTX);}
  Process -> (junction 12) [order 3] : ACK{Ack=Acknowledge(ACK.data.ID,ACK.data.RndLoss,ACK.data.RTR,ACK.data.Data,TX_ID,TX_RTR,TX_Data);}
  data: Status function_output; rx_id function_input double size=1; rx_loss function_input double size=1; Ack function_output; ack_id function_input double size=1; ack_loss function_input double size=1; ack_rtr function_input double size=1; ack_data function_input double size=1; tx_id function_input double size=1; tx_rtr function_input double size=1; tx_data function_input double size=1; TX input Bus: CAN_Message; ACK input Bus: CAN_Message; RX input Bus: CAN_Message; S local; Ack local; TX_ID local; TX_RTR local; TX_Data local; Port output; Success output; ReTX output

== matlab function NCS_Library/Network/CAN/CAN Node 4/Reception Control/Acknowledge/MATLAB Function ==
  data: ID0 input; ACK output; RTR0 input; Data0 input; ID1 input; RTR1 input; Data1 input; Loss input
function ACK = fcn(ID0,RTR0,Data0,ID1,RTR1,Data1,Loss)
% Compare the message ID, RTR, Data fields to acknowledge a successful send

if (ID0 == ID1 && RTR0 == RTR1 && Data0 == Data1 && Loss < 1)
    ACK = 1;
else
    ACK = 0;
end

== stateflow chart NCS_Library/Network/CAN/Logik/Slow_to_Fast/Switch_Logic ==
  settings: enableNonTerminalStates=1
  state Wait
    % Create Signal
    % for Switch
  (default) -> Wait
  Wait -> Wait [order 2] : Entity_out{path.data = 2; send(path)}
  Wait -> Wait [order 1] : Entity_in{path.data = 1; send(path)}
  data: Entity_in input; Entity_out input; path output

== matlab function NCS_Library/Network/ETB/Burst Device/Protocl Stack/TRDP PD/Simulink Function1/MATLAB Function ==
  data: Reply input; Address output; Source input
function Address = GetAddress(Reply, Source)
Address = Reply;
if Reply(1) == 0
    Address = Source;
end

== matlab function NCS_Library/Network/ETB/Burst Device/Protocl Stack/TRDP PD/Simulink Function1/MATLAB Function2 ==
  data: msgType input; ReplyAddress input; DestinationPull output
function DestinationPull = Receive(msgType, ReplyAddress)

DestinationPull = uint16( [0 0 0 0] );

if msgType == 11
    % Request
    DestinationPull = ReplyAddress;
end
        
end % end function

== matlab function NCS_Library/Controller/Controller/MATLAB Function1 ==
  data: Y_M input; U output
function U = Neg(Y_M)

Y_M(1,1) = -Y_M(1,1);
U = -Y_M;

end

== matlab function NCS_Library/Network/Gateway/Gateway1/Ethernet Interface/Subsystem4/MATLAB Function ==
  data: Data input; NEW output; Change input
function NEW = DetectNewData(Data, Change)

NEW = 0;
changed = 0;
for i=1:3
    for j=1:20
        if Change(i,j) ~= 0
            changed = 1;
            break;
        end
    end
end
        
if changed
    if Data(1,1) < 2
        % Data is empty
        NEW = 0;
    else
        % New Data
        NEW = Data(1,1)-1;
    end
end

end

== stateflow chart NCS_Library/Network/Gateway/Gateway1/Ethernet Interface/Subsystem4/Chart ==
  state Buffer_empty
    en: n=0;
    en: Push = 0;
  state Buffer_full
    du: Push=0;
  (default) -> Buffer_empty
  Buffer_full -> Buffer_empty [order 4] : [n==0]
  Buffer_empty -> Buffer_full [order 1] : [NEW>0]{n=n+NEW;}
  Buffer_empty -> Buffer_full [order 2] : [n>0]
  Buffer_full -> Buffer_full [order 1] : [NEW>0&&TIME==1]{n=n+NEW-1;}
  Buffer_full -> Buffer_full [order 3] : [TIME==1]{n=n-1;Push=1;}
  Buffer_full -> Buffer_full [order 2] : [NEW>0]{n=n+NEW}
  data: TIME input; n local; NEW input; Push output

== matlab function NCS_Library/Controller/Train Controller with PID/MATLAB Function ==
  data: Y_M input; v output
function v = fcn(Y_M)
%% Compute v
% This function computes the mean value for the velocity of the matrix Y_M
% received by several sensors

%% Init 
v = 0;
n_values = 0;

%% Compute v

% get n_values
for i = 1:length(Y_M)
    if Y_M(2,i) ~= 0
        n_values = n_values+1;
    end
end

% compute mean velocity
if n_values > 0
    v = sum(Y_M(2,:)) / n_values;
end

end % end function

== matlab function NCS_Library/Controller/Train Controller with PID/MATLAB Function1 ==
  data: u input; U output
function U = fcn(u)

U = zeros(3,20);
U(:,2) = u;

if u(1) ~= 0 || u(2) ~= 0 || u(3) ~= 0
    U(1,1) = 2;
else
    U(1,1) = 1;
end

end

== matlab function NCS_Library/Network/Applications/Multiplexer/Demux ==
  data: in input; U output; Y_M output
function [U, Y_M ] = Demux(in)

U = in(:,21:24);
Y_M = in(:,1:20);

== matlab function NCS_Library/Network/Applications/Multiplexer/Demux CAN ==
  data: U input; u1 output; u2 output; u3 output; u4 output
function [ u1, u2, u3, u4 ] = DemuxCAN(U)

u1 = U(:,1);
u2 = U(:,2);
u3 = U(:,3);
u4 = U(:,4);
